simulink model "data_memory1"  (Simulink 4.00)
settings: Solver=ode45  StartTime=0.0  StopTime=10.0  RelTol=1e-3
settings Model: LastModifiedBy=Administrator  BlockReductionOpt=off

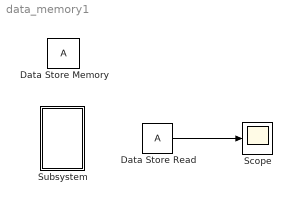
== system data_memory1 ==
  Data Store Memory : DataStoreMemory  DataStoreName=A  InitialValue=0
  Data Store Read : DataStoreRead  DataStoreName=A  SampleTime=0
  Scope : Scope
      settings: TimeRange=auto  YMin=-5  YMax=5  SaveToWorkspace=off  SaveName=ScopeData  LimitDataPoints=on  MaxDataPoints=5000
  Subsystem : Subsystem
      settings: RTWFcnNameOpts=Auto  RTWFileNameOpts=Auto
  wires:
  Data Store Read/1 -> Scope/1

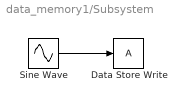
== system data_memory1/Subsystem ==
  Data Store Write : DataStoreWrite  DataStoreName=A  SampleTime=-1
  Sine Wave : Sin  Amplitude=1  Frequency=1  Phase=0  SampleTime=0
  wires:
  Sine Wave/1 -> Data Store Write/1
